simulink model "addgf2_test"  (R2020b)
settings: Solver=FixedStepAuto  StartTime=0.0  StopTime=inf  RelTol=1e-3
settings Model: SILPILModeSetting=veronly  ExtModeTrigDuration=2  Creator=tcbir  LastModifiedBy=tcbir
settings OptimizationCC: EnhancedBackFolding=on  PassReuseOutputArgsAs=Individual arguments  ZeroExternalMemoryAtStartup=off  ZeroInternalMemoryAtStartup=off  MaxStackSize=64  OptimizeBlockOrder=speed  DifferentSizesBufferReuse=on  OptimizationCustomize=off  EfficientTunableParamExpr=on
settings DebuggingCC: ParameterTunabilityLossMsg=error
settings HardwareCC: ProdBitPerInt=16  ProdBitPerPointer=16  ProdBitPerSizeT=16  ProdBitPerPtrDiffT=16  ProdLargestAtomicFloat=None  ProdWordSize=8  ProdHWDeviceType=Atmel->AVR  UseEmbeddedCoderFeatures=off  UseSimulinkCoderFeatures=off
settings RTWCC: Description=Embedded Coder  SystemTargetFile=ert.tlc  HardwareBoard=Arduino Mega 2560  TemplateMakefile=ert_default_tmf  Toolchain=Arduino AVR
settings CodeAppCC: ForceParamTrailComments=on  IgnoreCustomStorageClasses=off  OperatorAnnotations=on  SimulinkDataObjDesc=on  SFDataObjDesc=on  InsertBlockDesc=on
settings ERTTargetCC: SupportContinuousTime=on  SupportNonInlinedSFcns=on  SupportVariableSizeSignals=on  ExtModeStaticAllocSize=2048

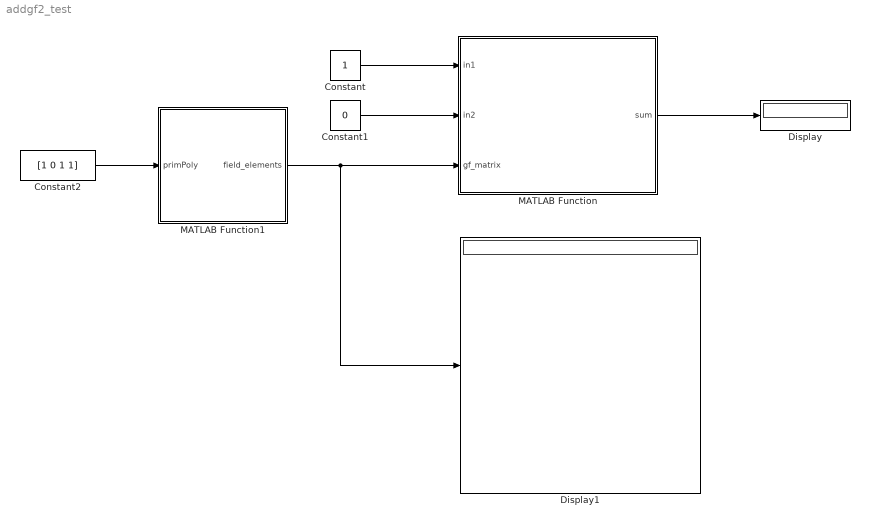
== system addgf2_test ==
  Constant : Constant
  Constant1 : Constant  Value=0
  Constant2 : Constant  Value=[1 0 1 1]
  Display : Display
  Display1 : Display
  MATLAB Function : MATLAB Function  TreatAsAtomicUnit=on
  MATLAB Function1 : MATLAB Function  TreatAsAtomicUnit=on
  wires:
  MATLAB Function1/1(field_elements) -> Display1/1, MATLAB Function/3(gf_matrix)
  Constant2/1 -> MATLAB Function1/1(primPoly)
  Constant/1 -> MATLAB Function/1(in1)
  Constant1/1 -> MATLAB Function/2(in2)
  MATLAB Function/1(sum) -> Display/1

== matlab function addgf2_test/MATLAB Function ==
  data: in1 input; sum output; in2 input; gf_matrix input
%adds two elements of the Galois Field
%in1, in2 are binary coefficients of alpha powers, LSB on right
%sum is power notation
function sum  = AddGF2m(in1, in2, gf_matrix)
m = numel(gf_matrix(1,:));
%convert power notation to rectangular
if in1 == -1
    sum = in2;
elseif in2 == -1
    sum = in1;
elseif in1 == in2
    sum = -1; %changed
else
    % had to put this sum = 0 here bacsue simulink whines about sum not
    % begin initialized in some decision trees
    sum = 0;
    gfIndx = in1 + 2; %account for inf and indexing
    r_in1 = gf_matrix(gfIndx, :);

    if in2 == -1
        r_in2 = zeros(1, m);
    else
        gfIndx = in2 + 2; %account for inf and indexing
        r_in2 = gf_matrix(gfIndx, :);
    end

    xor_res = xor(r_in1, r_in2); %xor the rectangular coordinates
    [rows, ~] = size(gf_matrix);

    for i = 1:rows %check each row of GF for matches
        if xor_res(1,:) == gf_matrix(i,:)
            if i == 1
                sum = -1;
            else
                sum = i - 2;%reverse indexing from above
            end
            break;
        end
    end
end 
end

== matlab function addgf2_test/MATLAB Function1 ==
  data: primPoly input; field_elements output
% GenerateGF2m: generates the selected Galois Field element. The inputs should be the
% order m and the coefficients of an appropriate primitive polynomial. The generated field,
% in either binary or power notation, may be a calling parameter for each of the other
% functions. Hint: I strongly suggest that you input the coefficients in “power” notation,
% with the highest order power on the left

function field_elements  = GenerateGF2m(primPoly) %primPoly in power notation, highest order on left

m = 3;
% hard coded size of retrun matrices and gf mtrix because simulink
% whines about variable output size. Havent figured out how to fix it
% ask laberge
gf = zeros(8, 3); %there are 2^m field elements
field_elements = zeros(8, 3); %there are 2^m field elements

gfIndx = 2; %gfIndx(1) holds initial state 
numShifts = (2^m) - 1;
s_reg = zeros(1,int8(m));
s_reg(end) = 1; %rightmost element of init shr is 1
gf(1, :) = 0;%write the contents of the init shift register to the matrix of gf elements
gf(2, :) = s_reg;
for i = 2:numShifts %number of shifts corresponds to power of primitive element
    carryOut = s_reg(1);%save the value to be wrapped
    for i0 = 1:numel(s_reg)-1
        if primPoly(i0 + 1) == 1
            s_reg(i0) = xor(carryOut, s_reg(i0 + 1));
        else
            s_reg(i0) = s_reg(i0 + 1);
        end
    end
    s_reg(end) = carryOut;
    gf(i+1,:) = s_reg; %add the newly shifted register to the gf matrix
end
field_elements = gf;
end
